simulink model "Input_Event"  (R2024a)
settings: Solver=FixedStepDiscrete  StartTime=0.0  StopTime=10.0  RelTol=1e-3
settings Model: Creator=VICTUS  LastModifiedBy=VICTUS

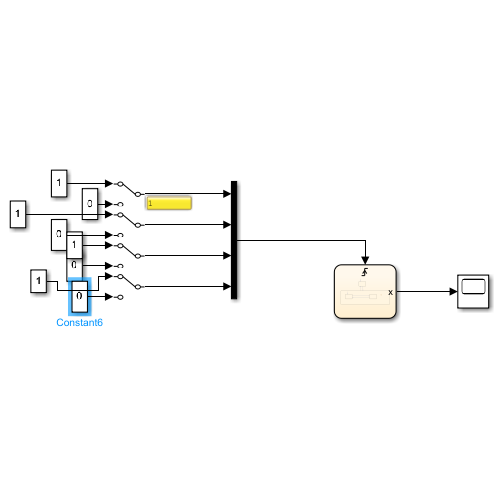
[thumbnail: Simulink's stored preview of the top-level diagram]
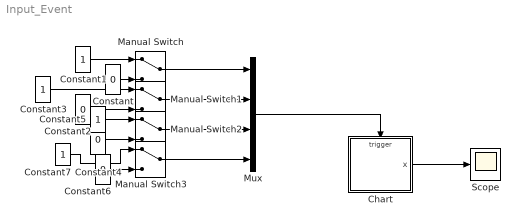
== system Input_Event ==
  Chart : Stateflow chart  TreatAsAtomicUnit=on
  Constant{,2,4,6} (4 alike) : Constant  Value=0
  Constant{1,3,5,7} (4 alike) : Constant
  Manual Switch{,1..3} (4 alike) : ManualSwitch
  Mux : Mux
  Scope : Scope
  wires:
  Mux/1 -> Chart/Trigger
  Manual Switch/1 -> Mux/1
  Manual Switch1/1 -> Mux/2
  Manual Switch2/1 -> Mux/3
  Constant/1 -> Manual Switch/2
  Constant1/1 -> Manual Switch/1
  Constant3/1 -> Manual Switch1/1
  Constant2/1 -> Manual Switch1/2
  Constant4/1 -> Manual Switch2/2
  Constant5/1 -> Manual Switch2/1
  Constant7/1 -> Manual Switch3/1
  Constant6/1 -> Manual Switch3/2
  Chart/1(x) -> Scope/1
  Manual Switch3/1 -> Mux/4

== stateflow chart Input_Event/Chart ==
  settings: executeAtInitialization=1
  state OFF
  state ON
    (history)
    state S1
      en:
      x = 5;
    state S2
      en:
      x = 10;
    (default) -> S1
    S1 -> S2 : S2
    S2 -> S1 : S1
  (default) -> OFF
  ON -> OFF : OFF
  OFF -> ON : ON
  data: x output
  events: S1 input RISING_EDGE_EVENT; S2 input RISING_EDGE_EVENT; ON input RISING_EDGE_EVENT; OFF input RISING_EDGE_EVENT
